simulink model "Traffic_lights_R2020a"  (R2020a)
settings: Solver=FixedStepAuto  StartTime=0.0  StopTime=10.0  MaxStep=1e-3  RelTol=1e-3  EnableMultiTasking=on
libraries: arduinolib x6
settings Model: SILPILModeSetting=veronly  ExtModeTrigDuration=2  Creator=hp  LastModifiedBy=hp
settings OptimizationCC: EnhancedBackFolding=on  PassReuseOutputArgsAs=Individual arguments  ZeroExternalMemoryAtStartup=off  ZeroInternalMemoryAtStartup=off  MaxStackSize=64  OptimizeBlockOrder=speed  DifferentSizesBufferReuse=on  OptimizationCustomize=off  EfficientTunableParamExpr=on
settings DebuggingCC: ParameterTunabilityLossMsg=error  UnconnectedInputMsg=none  UnconnectedOutputMsg=none  UnconnectedLineMsg=none
settings HardwareCC: ProdBitPerInt=16  ProdBitPerPointer=16  ProdBitPerSizeT=16  ProdBitPerPtrDiffT=16  ProdLargestAtomicFloat=None  ProdWordSize=8  ProdHWDeviceType=Atmel->AVR
settings ModelReferenceCC: EnableRefExpFcnMdlSchedulingChecks=off
settings SFSimCC: MATLABDynamicMemAlloc=off
settings RTWCC: SystemTargetFile=ert.tlc  HardwareBoard=Arduino Uno  TLCOptions=-aInlineSetEventsForThisBaseRateFcn=TLC_FALSE -aSuppressMultiTaskScheduler=TLC_FALSE -aRateBasedStepFcn=1  TemplateMakefile=ert_default_tmf  Toolchain=Arduino AVR  BuildConfiguration=Faster Runs
settings CodeAppCC: ForceParamTrailComments=on  IgnoreCustomStorageClasses=off  OperatorAnnotations=on  SimulinkDataObjDesc=on  SFDataObjDesc=on  InsertBlockDesc=on
settings ERTTargetCC: SupportContinuousTime=on  SupportVariableSizeSignals=on  ExtModeTransport=3  ExtModeStaticAlloc=on  ExtModeStaticAllocSize=250  ExtModeMexFile=ext_xcp  ExtModeIntrfLevel=Level2 - Open

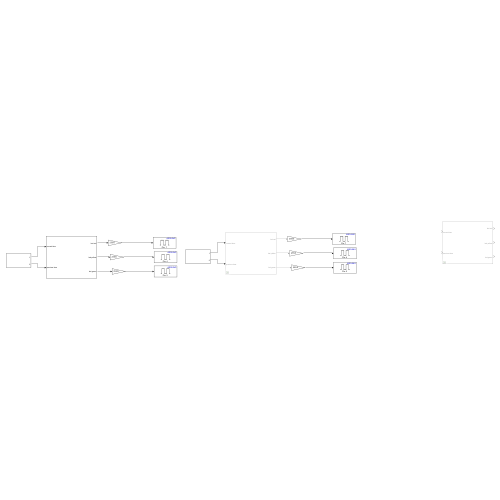
[thumbnail: Simulink's stored preview of the top-level diagram]
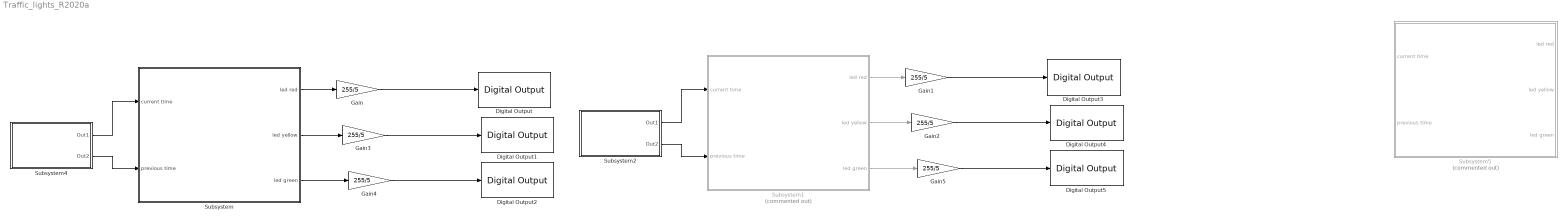
== system Traffic_lights_R2020a ==
  Digital Output : arduinolib/Digital Output  pinNumber=7  Direction=output  blockPlatform=arduino
  Digital Output1 : arduinolib/Digital Output  pinNumber=4  Direction=output  blockPlatform=arduino
  Digital Output2 : arduinolib/Digital Output  pinNumber=2  Direction=output  blockPlatform=arduino
  Digital Output3 : arduinolib/Digital Output  pinNumber=7  Direction=output  blockPlatform=arduino
  Digital Output4 : arduinolib/Digital Output  pinNumber=4  Direction=output  blockPlatform=arduino
  Digital Output5 : arduinolib/Digital Output  pinNumber=2  Direction=output  blockPlatform=arduino
  Gain{,1..5} (6 alike) : Gain  Gain=255/5
  Subsystem : Subsystem
  Subsystem1 : Subsystem  Commented=on
  Subsystem2 : Subsystem
  Subsystem4 : Subsystem
  Subsystem5 : Subsystem  Commented=on
  wires:
  Subsystem/1(led red) -> Gain/1
  Gain/1 -> Digital Output/1
  Subsystem/3(led green) -> Gain4/1
  Gain4/1 -> Digital Output2/1
  Gain3/1 -> Digital Output1/1
  Subsystem/2(led yellow) -> Gain3/1
  Subsystem4/1(Out1) -> Subsystem/1(current time)
  Subsystem4/2(Out2) -> Subsystem/2(previous time)
  Subsystem2/2(Out2) -> Subsystem1/2(previous time)
  Subsystem2/1(Out1) -> Subsystem1/1(current time)
  Subsystem1/2(led yellow) -> Gain2/1
  Gain2/1 -> Digital Output4/1
  Gain5/1 -> Digital Output5/1
  Subsystem1/3(led green) -> Gain5/1
  Gain1/1 -> Digital Output3/1
  Subsystem1/1(led red) -> Gain1/1

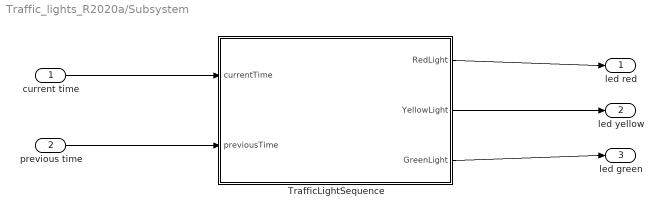
== system Traffic_lights_R2020a/Subsystem ==
  current time : Inport
  previous time : Inport  Port=2
  TrafficLightSequence : MATLAB Function  TreatAsAtomicUnit=on
  led red : Outport
  led yellow : Outport  Port=2
  led green : Outport  Port=3
  wires:
  current time/1 -> TrafficLightSequence/1(currentTime)
  previous time/1 -> TrafficLightSequence/2(previousTime)
  TrafficLightSequence/1(RedLight) -> led red/1
  TrafficLightSequence/2(YellowLight) -> led yellow/1
  TrafficLightSequence/3(GreenLight) -> led green/1

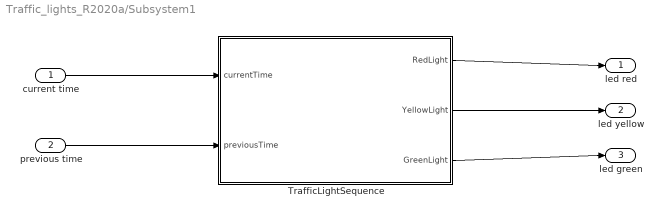
== system Traffic_lights_R2020a/Subsystem1 ==
  current time : Inport
  previous time : Inport  Port=2
  TrafficLightSequence : MATLAB Function  TreatAsAtomicUnit=on
  led red : Outport
  led yellow : Outport  Port=2
  led green : Outport  Port=3
  wires:
  TrafficLightSequence/3(GreenLight) -> led green/1
  TrafficLightSequence/2(YellowLight) -> led yellow/1
  TrafficLightSequence/1(RedLight) -> led red/1
  previous time/1 -> TrafficLightSequence/2(previousTime)
  current time/1 -> TrafficLightSequence/1(currentTime)

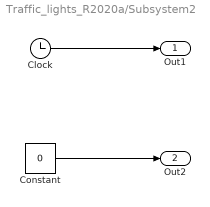
== system Traffic_lights_R2020a/Subsystem2 ==
  Clock : Clock
  Constant : Constant  Value=0
  Out1 : Outport
  Out2 : Outport  Port=2
  wires:
  Constant/1 -> Out2/1
  Clock/1 -> Out1/1

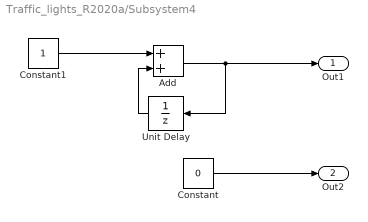
== system Traffic_lights_R2020a/Subsystem4 ==
  Add : Sum
  Constant : Constant  Value=0
  Constant1 : Constant
  Unit Delay : UnitDelay  SampleTime=2  HasFrameUpgradeWarning=on
  Out1 : Outport
  Out2 : Outport  Port=2
  wires:
  Constant/1 -> Out2/1
  Add/1 -> Unit Delay/1, Out1/1
  Constant1/1 -> Add/1
  Unit Delay/1 -> Add/2

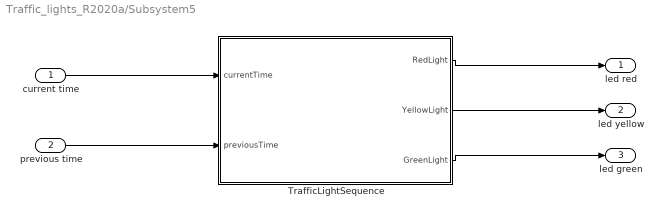
== system Traffic_lights_R2020a/Subsystem5 ==
  current time : Inport
  previous time : Inport  Port=2
  TrafficLightSequence : MATLAB Function  TreatAsAtomicUnit=on
  led red : Outport
  led yellow : Outport  Port=2
  led green : Outport  Port=3
  wires:
  TrafficLightSequence/3(GreenLight) -> led green/1
  TrafficLightSequence/2(YellowLight) -> led yellow/1
  TrafficLightSequence/1(RedLight) -> led red/1
  previous time/1 -> TrafficLightSequence/2(previousTime)
  current time/1 -> TrafficLightSequence/1(currentTime)

== matlab function Traffic_lights_R2020a/Subsystem5/TrafficLightSequence ==
  data: currentTime input; RedLight output; previousTime input; YellowLight output; GreenLight output
function [RedLight, YellowLight, GreenLight] = TrafficLightSequence(currentTime, previousTime)
    % Traffic light sequence with delays
    
    % Define timing parameters (in seconds)
    redTime = 10;
    yellowTime = 5;
    greenTime = 11;

    % Initialize outputs
    RedLight = 0;
    YellowLight = 0;
    GreenLight = 0;

    % Calculate elapsed time since the last update
    elapsedTime = currentTime - previousTime;

    % Traffic light sequence logic
    if elapsedTime >= redTime + yellowTime + greenTime
        % Reset the timer
        previousTime = currentTime;
    end

    if elapsedTime < redTime
        % Red light is ON
        RedLight = 1;
    elseif elapsedTime < redTime + yellowTime
        % Yellow light is ON
        YellowLight = 1;
    else
        % Green light is ON
        GreenLight = 1;
    end
end

== matlab function Traffic_lights_R2020a/Subsystem/TrafficLightSequence ==
  data: currentTime input; RedLight output; previousTime input; YellowLight output; GreenLight output
function [RedLight, YellowLight, GreenLight] = TrafficLightSequenceContinuous(currentTime, previousTime)
    % Continuous traffic light sequence
    
    % Adjust timing parameters (in seconds)
    redTime = 2;     % Set the duration for the red light
    yellowTime = 2;   % Set the duration for the yellow light
    greenTime = 2;   % Set the duration for the green light

    % Initialize outputs
    RedLight = 0;
    YellowLight = 0;
    GreenLight = 0;

    % Calculate elapsed time since the last update
    elapsedTime = currentTime - previousTime;

    % Calculate the time within a complete cycle
    cycleTime = redTime + yellowTime + greenTime;

    % Determine the current phase in the cycle
    currentPhase = mod(elapsedTime, cycleTime);

    % Traffic light sequence logic
    if currentPhase < redTime
        % Red light is ON
        RedLight = 1;
    elseif currentPhase < redTime + yellowTime
        % Yellow light is ON
        YellowLight = 1;
    else
        % Green light is ON
        GreenLight = 1;
    end
end

== matlab function Traffic_lights_R2020a/Subsystem1/TrafficLightSequence ==
  data: currentTime input; RedLight output; previousTime input; YellowLight output; GreenLight output
function [RedLight, YellowLight, GreenLight] = TrafficLightSequenceContinuous(currentTime, previousTime)
    % Continuous traffic light sequence
    
    % Adjust timing parameters (in seconds)
    redTime = 2;     % Set the duration for the red light
    yellowTime = 2;   % Set the duration for the yellow light
    greenTime = 2;   % Set the duration for the green light

    % Initialize outputs
    RedLight = 0;
    YellowLight = 0;
    GreenLight = 0;

    % Calculate elapsed time since the last update
    elapsedTime = currentTime - previousTime;

    % Calculate the time within a complete cycle
    cycleTime = redTime + yellowTime + greenTime;

    % Determine the current phase in the cycle
    currentPhase = mod(elapsedTime, cycleTime);

    % Traffic light sequence logic
    if currentPhase < redTime
        % Red light is ON
        RedLight = 1;
    elseif currentPhase < redTime + yellowTime
        % Yellow light is ON
        YellowLight = 1;
    else
        % Green light is ON
        GreenLight = 1;
    end
end
